simulink model "questao5"  (R2021b)
settings: Solver=VariableStepAuto  StartTime=0.0  StopTime=1800  RelTol=1e-3
values from neighbouring files (symbols this model uses):
  A = [A11 A12 ... (first row only)    [main.m]
  B = [Bu Bd]    [main.m]
  C = [1 0]    [main.m]
  D = zeros(1,4)    [main.m]
  dF = 0    [main.m]
  dFj2 = dFj*10    (= 0.000472)    [main.m]
  dTi = 0    [main.m]
  dTij = 0    [main.m]
  Fjs = 7.079e-4    (= 0.0007079)    [main.m]
  Fs = 4.720e-4    (= 0.000472)    [main.m]
  G = p*Bu    [main.m]
  Gd1 = p*[Bd11 ... (first row only)    [main.m]
  Gd2 = p*[Bd12 ... (first row only)    [main.m]
  Gd3 = p*[Bd13 ... (first row only)    [main.m]
  Tis = 10    [main.m]
  Tjis = 93.33    [main.m]
  Tjs = 65.56    [main.m]
  Ts = 51.67    [main.m]
settings Model: Creator=luang  LastModifiedBy=luang

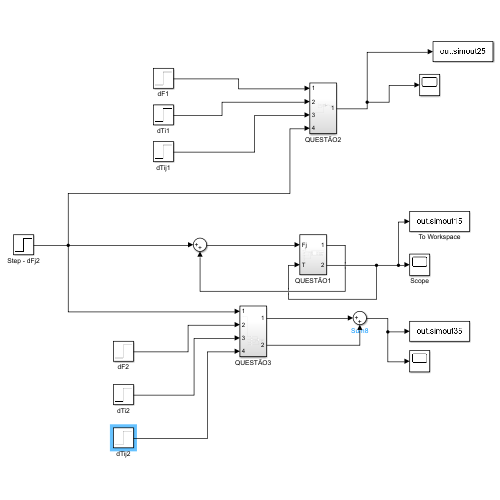
[thumbnail: Simulink's stored preview of the top-level diagram]
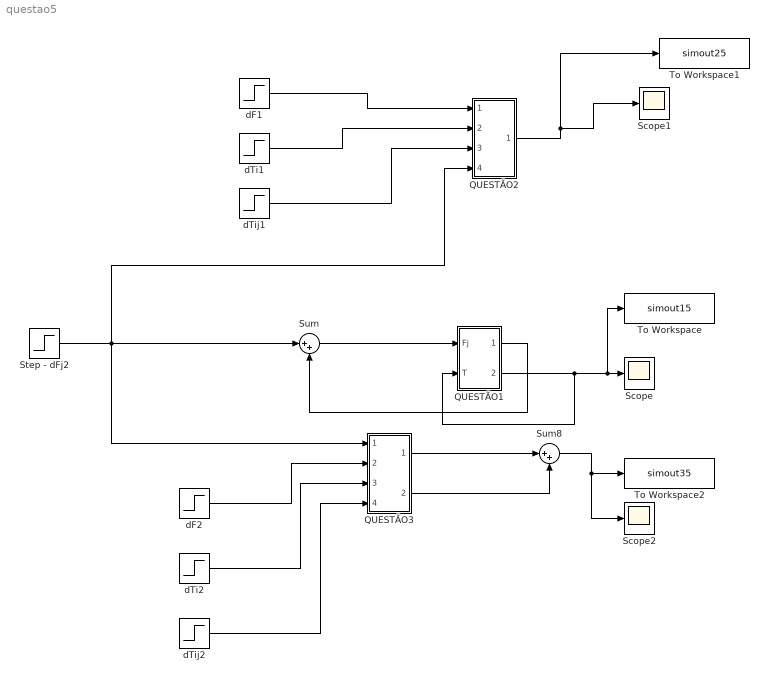
== system questao5 ==
  QUESTÃO1 : Subsystem
  QUESTÃO2 : Subsystem
  QUESTÃO3 : Subsystem
  Scope : Scope
  Scope1 : Scope
  Scope2 : Scope
  Step - dFj2 : Step  After=dFj2  SampleTime=0
  Sum : Sum  Inputs=|++
  Sum8 : Sum  Inputs=|++
  To Workspace : ToWorkspace  VariableName=simout15  SaveFormat=Structure With Time  SampleTime=-1
  To Workspace1 : ToWorkspace  VariableName=simout25  SaveFormat=Structure With Time  SampleTime=-1
  To Workspace2 : ToWorkspace  VariableName=simout35  SaveFormat=Structure With Time  SampleTime=-1
  dF1 : Step  After=dF  SampleTime=0
  dF2 : Step  After=dF  SampleTime=0
  dTi1 : Step  After=dTi  SampleTime=0
  dTi2 : Step  After=dTi  SampleTime=0
  dTij1 : Step  After=dTij  SampleTime=0
  dTij2 : Step  After=dTij  SampleTime=0
  wires:
  Step - dFj2/1 -> QUESTÃO3/1(In1), QUESTÃO2/4(In4), Sum/1
  Sum8/1 -> Scope2/1, To Workspace2/1
  QUESTÃO2/1(Out1) -> Scope1/1, To Workspace1/1
  dF1/1 -> QUESTÃO2/1(In1)
  dTi1/1 -> QUESTÃO2/2(In2)
  dTij1/1 -> QUESTÃO2/3(In3)
  QUESTÃO1/2(Out2) -> To Workspace/1, Scope/1, QUESTÃO1/2(T)
  Sum/1 -> QUESTÃO1/1(Fj)
  QUESTÃO1/1(Out1) -> Sum/2
  dF2/1 -> QUESTÃO3/2(In2)
  dTi2/1 -> QUESTÃO3/3(In3)
  dTij2/1 -> QUESTÃO3/4(In4)
  QUESTÃO3/1(Out1) -> Sum8/1
  QUESTÃO3/2(Out2) -> Sum8/2

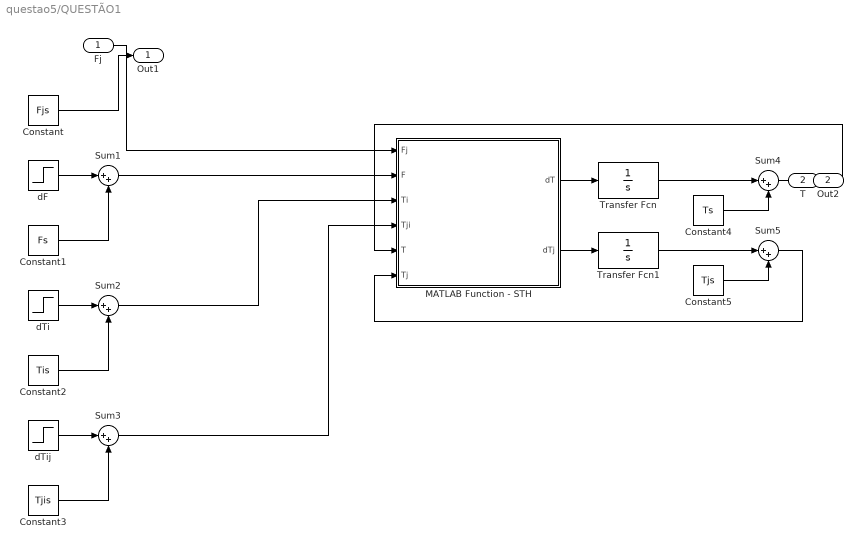
== system questao5/QUESTÃO1 ==
  Fj : Inport
  T : Inport  Port=2
  Constant : Constant  Value=Fjs
  Constant1 : Constant  Value=Fs
  Constant2 : Constant  Value=Tis
  Constant3 : Constant  Value=Tjis
  Constant4 : Constant  Value=Ts
  Constant5 : Constant  Value=Tjs
  MATLAB Function - STH : MATLAB Function  TreatAsAtomicUnit=on
  Sum{1..5} (5 alike) : Sum  Inputs=|++
  Transfer Fcn : TransferFcn  Denominator=[1 0]
  Transfer Fcn1 : TransferFcn  Denominator=[1 0]
  dF : Step  After=dF  SampleTime=0
  dTi : Step  After=dTi  SampleTime=0
  dTij : Step  After=dTij  SampleTime=0
  Out1 : Outport
  Out2 : Outport  Port=2
  wires:
  T/1 -> MATLAB Function - STH/5(T)
  Constant3/1 -> Sum3/2
  Transfer Fcn/1 -> Sum4/1
  Transfer Fcn1/1 -> Sum5/1
  Sum2/1 -> MATLAB Function - STH/3(Ti)
  MATLAB Function - STH/1(dT) -> Transfer Fcn/1
  Constant4/1 -> Sum4/2
  Sum5/1 -> MATLAB Function - STH/6(Tj)
  Fj/1 -> MATLAB Function - STH/1(Fj)
  dTij/1 -> Sum3/1
  Constant5/1 -> Sum5/2
  Sum1/1 -> MATLAB Function - STH/2(F)
  dF/1 -> Sum1/1
  Constant2/1 -> Sum2/2
  Sum3/1 -> MATLAB Function - STH/4(Tji)
  Constant1/1 -> Sum1/2
  MATLAB Function - STH/2(dTj) -> Transfer Fcn1/1
  dTi/1 -> Sum2/1
  Sum4/1 -> Out2/1
  Constant/1 -> Out1/1

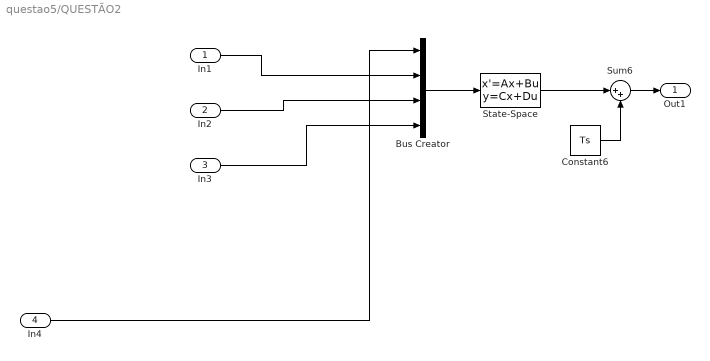
== system questao5/QUESTÃO2 ==
  In1 : Inport
  In2 : Inport  Port=2
  In3 : Inport  Port=3
  In4 : Inport  Port=4
  Bus Creator : BusCreator  Inputs=4
  Constant6 : Constant  Value=Ts
  State-Space : StateSpace  A=A  B=B  C=C  D=D  InitialCondition=0
  Sum6 : Sum  Inputs=|++
  Out1 : Outport
  wires:
  In3/1 -> Bus Creator/4
  Constant6/1 -> Sum6/2
  Sum6/1 -> Out1/1
  In2/1 -> Bus Creator/3
  State-Space/1 -> Sum6/1
  Bus Creator/1 -> State-Space/1
  In1/1 -> Bus Creator/2
  In4/1 -> Bus Creator/1

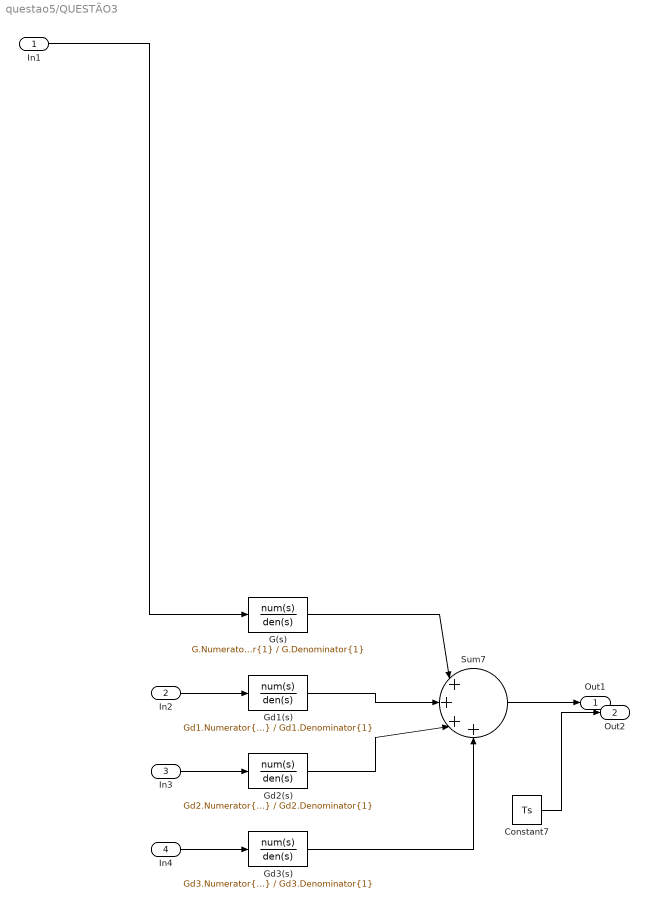
== system questao5/QUESTÃO3 ==
  In1 : Inport
  In2 : Inport  Port=2
  In3 : Inport  Port=3
  In4 : Inport  Port=4
  Constant7 : Constant  Value=Ts
  G(s) : TransferFcn  Numerator=G.Numerator{1}  Denominator=G.Denominator{1}
  Gd1(s) : TransferFcn  Numerator=Gd1.Numerator{1}  Denominator=Gd1.Denominator{1}
  Gd2(s) : TransferFcn  Numerator=Gd2.Numerator{1}  Denominator=Gd2.Denominator{1}
  Gd3(s) : TransferFcn  Numerator=Gd3.Numerator{1}  Denominator=Gd3.Denominator{1}
  Sum7 : Sum  Inputs=|++++
  Out1 : Outport
  Out2 : Outport  Port=2
  wires:
  Gd1(s)/1 -> Sum7/2
  Constant7/1 -> Out2/1
  G(s)/1 -> Sum7/1
  Gd2(s)/1 -> Sum7/3
  In1/1 -> G(s)/1
  In3/1 -> Gd2(s)/1
  Gd3(s)/1 -> Sum7/4
  In2/1 -> Gd1(s)/1
  Sum7/1 -> Out1/1
  In4/1 -> Gd3(s)/1

== matlab function questao5/QUESTÃO1/MATLAB Function - STH ==
  data: Fj input; dT output; F input; Ti input; Tji input; T input; Tj input; dTj output
function [dT, dTj] = fcn(Fj, F, Ti, Tji, T, Tj)

V = 283.168e-3;
UA = 3.065;
pcp = 2.165e3;
Vj = 28.319e-3;
pcpj = 2.165e3;

dT = (F/V)*(Ti - T) + (UA/(V*pcp))*(Tj - T);

dTj = (Fj/Vj)*(Tji - Tj) - ((UA/(Vj*pcpj))*(Tj - T));
